simulink model "exp3_q23"  (R2019a)
settings: Solver=FixedStepAuto  StartTime=0.0  StopTime=5e-1  FixedStep=1e-7  RelTol=1e-3
libraries: dsparch4 x2, simulink x1
settings Model: Creator=marco  LastModifiedBy=marco
settings DebuggingCC: SigSpecEnsureSampleTimeMsg=none

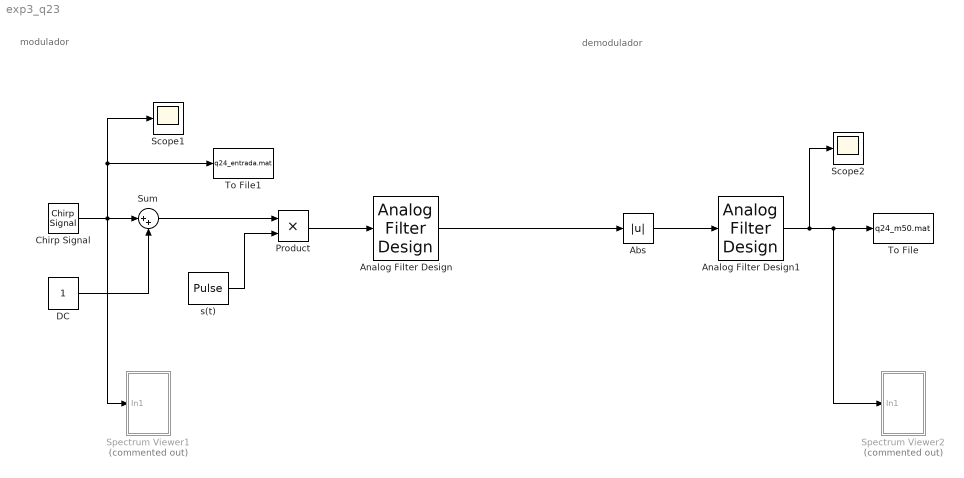
== system exp3_q23 ==
  note: demodulador
  note: modulador
  Abs : Abs
  Analog Filter Design : dsparch4/Analog Filter Design  method=Butterworth  filttype=Bandpass  N=10  Wlo=2*pi*980e3  Whi=2*pi*1020e3  Rp=2  Rs=40
  Analog Filter Design1 : dsparch4/Analog Filter Design  method=Butterworth  filttype=Lowpass  N=10  Wlo=2*pi*500e3  Whi=2*pi*1020e3  Rp=2  Rs=40
  Chirp Signal : simulink/Sources/Chirp Signal  f1=100  T=5e-1  f2=4e3
  DC : Constant
  Product : Product
  Scope1 : Scope
  Scope2 : Scope
  Spectrum Viewer1 : Subsystem  Commented=on
  Spectrum Viewer2 : Subsystem  Commented=on
  Sum : Sum  Inputs=|++
  To File : ToFile  Filename=q24_m50.mat  MatrixName=q24_m50  SaveFormat=Timeseries  SampleTime=1e-4
  To File1 : ToFile  Filename=q24_entrada.mat  MatrixName=q24_entrada  SaveFormat=Timeseries  SampleTime=1e-4
  "s(t) " : DiscretePulseGenerator  PulseType=Time based  Period=1e-6  PulseWidth=50
  wires:
  Product/1 -> Analog Filter Design/1
  Sum/1 -> Product/1
  Chirp Signal/1 -> To File1/1, Scope1/1, Spectrum Viewer1/1(In1), Sum/1
  DC/1 -> Sum/2
  "s(t) "/1 -> Product/2
  Analog Filter Design/1 -> Abs/1
  Abs/1 -> Analog Filter Design1/1
  Analog Filter Design1/1 -> To File/1, Spectrum Viewer2/1(In1), Scope2/1

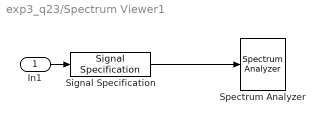
== system exp3_q23/Spectrum Viewer1 ==
  In1 : Inport
  Signal Specification : SignalSpecification  SampleTime=0.5e-5
  Spectrum Analyzer : SpectrumAnalyzer
  wires:
  In1/1 -> Signal Specification/1
  Signal Specification/1 -> Spectrum Analyzer/1

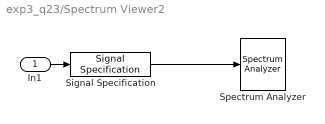
== system exp3_q23/Spectrum Viewer2 ==
  In1 : Inport
  Signal Specification : SignalSpecification  SampleTime=0.5e-5
  Spectrum Analyzer : SpectrumAnalyzer
  wires:
  In1/1 -> Signal Specification/1
  Signal Specification/1 -> Spectrum Analyzer/1
